simulink library "Pendel_Control"  (R2017b)
settings: Solver=VariableStepAuto  StartTime=0.0  StopTime=10.0  RelTol=1e-3
undefined symbols (not defined in the file): Angular2Linear, DiscIntNeverNeededParam, g, l, m, Ref_Bottom, Reset_Position_Bottom, SwitchAngle, U_Bottom
libraries: simulink x12, cstblocks x2
settings Model: Creator=BIROMED  LastModifiedBy=BIROMED

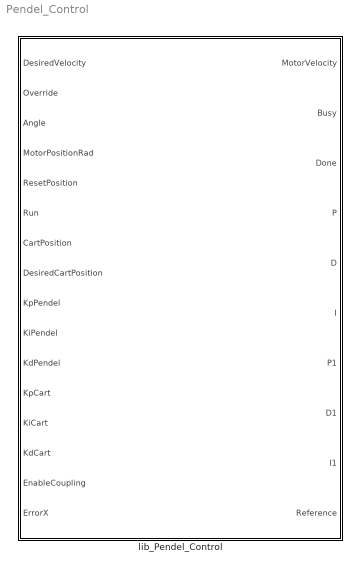
== system Pendel_Control ==
  lib_Pendel_Control : Subsystem

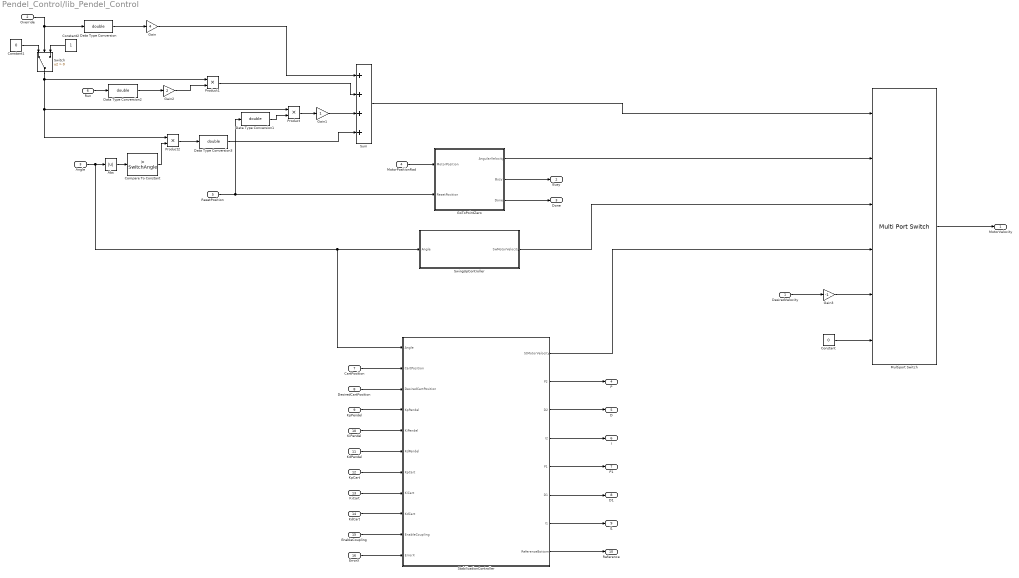
== system Pendel_Control/lib_Pendel_Control ==
  DesiredVelocity : Inport  OutDataTypeStr=double
  Override : Inport  Port=2  OutDataTypeStr=boolean
  Angle : Inport  Port=3
  MotorPositionRad : Inport  Port=4
  ResetPosition : Inport  Port=5  OutDataTypeStr=boolean
  Run : Inport  Port=6
  CartPosition : Inport  Port=7
  DesiredCartPosition : Inport  Port=8
  KpPendel : Inport  Port=9
  KiPendel : Inport  Port=10
  KdPendel : Inport  Port=11
  KpCart : Inport  Port=12  OutDataTypeStr=double
  KiCart : Inport  Port=13  OutDataTypeStr=double
  KdCart : Inport  Port=14  OutDataTypeStr=double
  EnableCoupling : Inport  Port=15  OutDataTypeStr=boolean
  ErrorX : Inport  Port=16  OutDataTypeStr=double
  Abs : Abs
  Compare To Constant : simulink/Logic and Bit Operations/Compare To Constant  relop=>  const=SwitchAngle  OutDataTypeStr=boolean
  Constant : Constant  Value=0
  Constant1 : Constant  Value=0
  Constant2 : Constant
  Data Type Conversion{,1..3} (4 alike) : DataTypeConversion  OutDataTypeStr=double
  Gain : Gain  Gain=4
  Gain1 : Gain
  Gain2 : Gain  Gain=2
  Gain3 : Gain  Gain=-1
  GoToPointZero : Subsystem
  Multiport Switch : MultiPortSwitch  Inputs=5
  Product : Product
  Product1 : Product
  Product2 : Product
  StabilizationController : Subsystem
  Sum : Sum  Inputs=++++
  SwingUpController : Subsystem
  Switch : Switch  Criteria=u2 > Threshold
  MotorVelocity : Outport
  Busy : Outport  Port=2  OutDataTypeStr=boolean
  Done : Outport  Port=3  OutDataTypeStr=boolean
  P : Outport  Port=4
  D : Outport  Port=5
  I : Outport  Port=6
  P1 : Outport  Port=7
  D1 : Outport  Port=8
  I1 : Outport  Port=9
  Reference : Outport  Port=10
  wires:
  KpCart/1 -> StabilizationController/7(KpCart)
  KpPendel/1 -> StabilizationController/4(KpPendel)
  EnableCoupling/1 -> StabilizationController/10(EnableCoupling)
  Data Type Conversion3/1 -> Sum/4
  KiPendel/1 -> StabilizationController/5(KiPendel)
  Data Type Conversion/1 -> Gain/1
  Gain3/1 -> Multiport Switch/5
  Product/1 -> Gain1/1
  StabilizationController/4(I2) -> I/1
  Gain2/1 -> Product1/2
  ResetPosition/1 -> GoToPointZero/2(ResetPosition), Data Type Conversion1/1
  Product1/1 -> Sum/2
  Override/1 -> Data Type Conversion/1, Switch/2
  GoToPointZero/2(Busy) -> Busy/1
  CartPosition/1 -> StabilizationController/2(CartPosition)
  StabilizationController/7(I1) -> I1/1
  Abs/1 -> Compare To Constant/1
  GoToPointZero/1(AngularVelocity) -> Multiport Switch/2
  DesiredCartPosition/1 -> StabilizationController/3(DesiredCartPosition)
  KiCart/1 -> StabilizationController/8(KiCart)
  Gain1/1 -> Sum/3
  Switch/1 -> Product1/1, Product2/1, Product/1
  StabilizationController/8(ReferenceBottom) -> Reference/1
  Product2/1 -> Data Type Conversion3/1
  Constant2/1 -> Switch/3
  Data Type Conversion2/1 -> Gain2/1
  Constant1/1 -> Switch/1
  Run/1 -> Data Type Conversion2/1
  Compare To Constant/1 -> Product2/2
  SwingUpController/1(SwMotorVelocity) -> Multiport Switch/3
  ErrorX/1 -> StabilizationController/11(ErrorX)
  Angle/1 -> StabilizationController/1(Angle), SwingUpController/1(Angle), Abs/1
  StabilizationController/6(D1) -> D1/1
  Sum/1 -> Multiport Switch/1
  StabilizationController/1(StMotorVelocity) -> Multiport Switch/4
  KdPendel/1 -> StabilizationController/6(KdPendel)
  Constant/1 -> Multiport Switch/6
  StabilizationController/3(D2) -> D/1
  StabilizationController/2(P2) -> P/1
  Gain/1 -> Sum/1
  DesiredVelocity/1 -> Gain3/1
  Multiport Switch/1 -> MotorVelocity/1
  KdCart/1 -> StabilizationController/9(KdCart)
  MotorPositionRad/1 -> GoToPointZero/1(MotorPosition)
  StabilizationController/5(P1) -> P1/1
  Data Type Conversion1/1 -> Product/2
  GoToPointZero/3(Done) -> Done/1

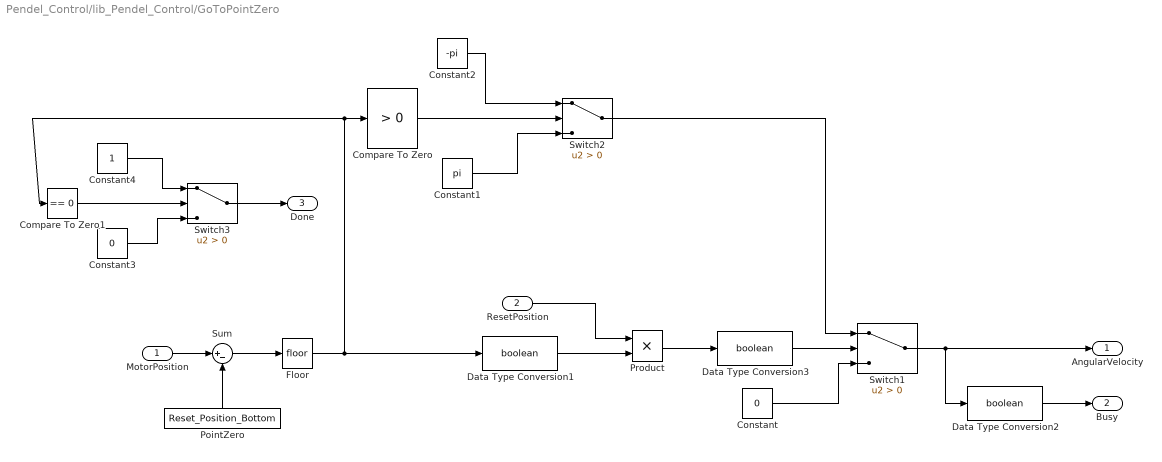
== system Pendel_Control/lib_Pendel_Control/GoToPointZero ==
  MotorPosition : Inport
  ResetPosition : Inport  Port=2
  Compare To Zero : simulink/Logic and Bit Operations/Compare To Zero  relop=>  OutDataTypeStr=boolean
  Compare To Zero1 : simulink/Logic and Bit Operations/Compare To Zero  relop===  OutDataTypeStr=boolean
  Constant : Constant  Value=0
  Constant1 : Constant  Value=pi
  Constant2 : Constant  Value=-pi
  Constant3 : Constant  Value=0
  Constant4 : Constant
  Data Type Conversion1 : DataTypeConversion  OutDataTypeStr=boolean
  Data Type Conversion2 : DataTypeConversion  OutDataTypeStr=boolean
  Data Type Conversion3 : DataTypeConversion  OutDataTypeStr=boolean
  Floor : Rounding
  PointZero : Constant  Value=Reset_Position_Bottom
  Product : Product
  Sum : Sum  Inputs=|+-
  Switch1 : Switch  Criteria=u2 > Threshold  OutDataTypeStr=double
  Switch2 : Switch  Criteria=u2 > Threshold
  Switch3 : Switch  Criteria=u2 > Threshold  OutDataTypeStr=boolean
  AngularVelocity : Outport
  Busy : Outport  Port=2
  Done : Outport  Port=3
  wires:
  Switch1/1 -> Data Type Conversion2/1, AngularVelocity/1
  PointZero/1 -> Sum/2
  Floor/1 -> Data Type Conversion1/1, Compare To Zero1/1, Compare To Zero/1
  MotorPosition/1 -> Sum/1
  Sum/1 -> Floor/1
  Constant/1 -> Switch1/3
  Compare To Zero/1 -> Switch2/2
  Constant1/1 -> Switch2/3
  Constant2/1 -> Switch2/1
  Switch2/1 -> Switch1/1
  Data Type Conversion2/1 -> Busy/1
  Data Type Conversion3/1 -> Switch1/2
  Constant3/1 -> Switch3/3
  Switch3/1 -> Done/1
  Constant4/1 -> Switch3/1
  Compare To Zero1/1 -> Switch3/2
  Product/1 -> Data Type Conversion3/1
  Data Type Conversion1/1 -> Product/2
  ResetPosition/1 -> Product/1

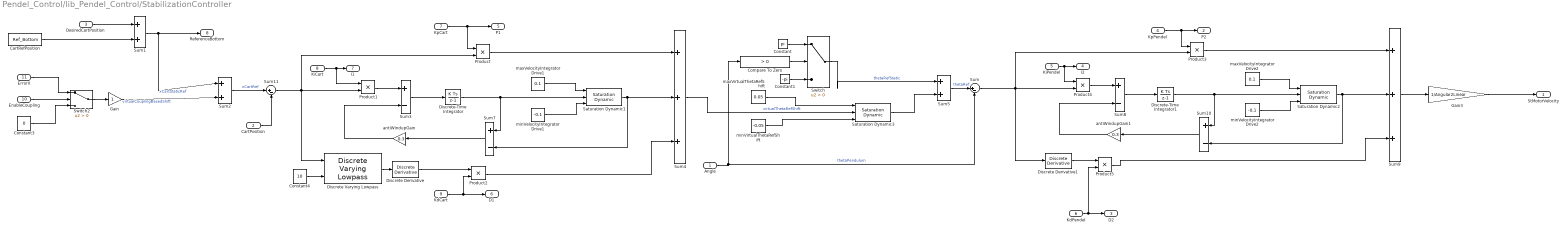
== system Pendel_Control/lib_Pendel_Control/StabilizationController ==
  Angle : Inport
  CartPosition : Inport  Port=2
  DesiredCartPosition : Inport  Port=3
  KpPendel : Inport  Port=4
  KiPendel : Inport  Port=5
  KdPendel : Inport  Port=6
  KpCart : Inport  Port=7
  KiCart : Inport  Port=8
  KdCart : Inport  Port=9
  EnableCoupling : Inport  Port=10
  ErrorX : Inport  Port=11
  CartRefPosition : Constant  Value=Ref_Bottom
  Compare To Zero : simulink/Logic and Bit Operations/Compare To Zero  relop=>  OutDataTypeStr=boolean
  Constant : Constant  Value=pi
  Constant1 : Constant  Value=-pi
  Constant3 : Constant  Value=0
  Constant4 : Constant  Value=10
  Discrete Derivative : simulink/Discrete/Discrete Derivative  gainval=1.0  ICPrevScaledInput=0.0  OutMin=[]  OutMax=[]  OutDataType=fixdt(1, 16)  OutScaling=2^-10  DoSatur=off
  Discrete Derivative1 : simulink/Discrete/Discrete Derivative  gainval=1.0  ICPrevScaledInput=0.0  OutMin=[]  OutMax=[]  OutDataType=fixdt(1, 16)  OutScaling=2^-10  DoSatur=off
  Discrete Varying Lowpass : cstblocks/Linear Parameter Varying/Discrete Varying Lowpass  N=1  w0=0  Ts=0.001
      settings: SourceProductName=Control System Toolbox  SourceProductBaseCode=CT
  Discrete-Time Integrator : DiscreteIntegrator  InitialConditionSetting=State (most efficient)  SampleTime=-1  ICPrevOutput=DiscIntNeverNeededParam  ICPrevScaledInput=DiscIntNeverNeededParam
  Discrete-Time Integrator1 : DiscreteIntegrator  InitialConditionSetting=State (most efficient)  SampleTime=-1  ICPrevOutput=DiscIntNeverNeededParam  ICPrevScaledInput=DiscIntNeverNeededParam
  Gain : Gain
  Gain3 : Gain  Gain=1/Angular2Linear
  Product{,1..5} (6 alike) : Product
  Saturation Dynamic1 : simulink/Discontinuities/Saturation Dynamic  OutMin=[]  OutMax=[]  OutDataTypeStr=Inherit: Same as second input  OutDataType=fixdt(1, 16)  OutScaling=2^-10  DoSatur=off
  Saturation Dynamic2 : simulink/Discontinuities/Saturation Dynamic  OutMin=[]  OutMax=[]  OutDataTypeStr=Inherit: Same as second input  OutDataType=fixdt(1, 16)  OutScaling=2^-10  DoSatur=off
  Saturation Dynamic3 : simulink/Discontinuities/Saturation Dynamic  OutMin=[]  OutMax=[]  OutDataTypeStr=Inherit: Same as second input  OutDataType=fixdt(1, 16)  OutScaling=2^-10  DoSatur=off
  Sum : Sum  Inputs=|+-
  Sum1 : Sum
  Sum{3,7..8,10} (4 alike) : Sum  Inputs=+-
  Sum11 : Sum  Inputs=|+-
  Sum2 : Sum  Inputs=|++
  Sum4 : Sum  Inputs=+++
  Sum5 : Sum  Inputs=|++
  Sum9 : Sum  Inputs=+++
  Switch : Switch  Criteria=u2 > Threshold
  Switch2 : Switch  Criteria=u2 > Threshold
  antiWindupGain : Gain  Gain=0.3
  antiWindupGain1 : Gain  Gain=0.3
  maxVelocityIntegratorDrive1 : Constant  Value=0.1
  maxVelocityIntegratorDrive2 : Constant  Value=0.1
  maxVirtualThetaRefShift : Constant  Value=0.05
  minVelocityIntegratorDrive1 : Constant  Value=-0.1
  minVelocityIntegratorDrive2 : Constant  Value=-0.1
  minVirtualThetaRefShift : Constant  Value=-0.05
  StMotorVelocity : Outport
  P2 : Outport  Port=2
  D2 : Outport  Port=3
  I2 : Outport  Port=4
  P1 : Outport  Port=5
  D1 : Outport  Port=6
  I1 : Outport  Port=7
  ReferenceBottom : Outport  Port=8
  wires:
  Sum5/1 -> Sum/1  "thetaRef"
  Compare To Zero/1 -> Switch/2
  CartPosition/1 -> Sum11/2
  KpPendel/1 -> Product3/1, P2/1
  KiPendel/1 -> Product4/1, I2/1
  KdPendel/1 -> Product5/2, D2/1
  KpCart/1 -> Product/1, P1/1
  KdCart/1 -> Product2/2, D1/1
  Gain3/1 -> StMotorVelocity/1
  Angle/1 -> Compare To Zero/1, Sum/2  "thetaPendulum"
  Constant/1 -> Switch/1
  Constant1/1 -> Switch/3
  KiCart/1 -> Product1/1, I1/1
  Sum9/1 -> Gain3/1
  Discrete-Time Integrator/1 -> Sum7/1, Saturation Dynamic1/2
  Sum11/1 -> Discrete Varying Lowpass/1, Product1/2, Product/2
  Sum3/1 -> Discrete-Time Integrator/1
  Sum7/1 -> antiWindupGain/1
  antiWindupGain/1 -> Sum3/2
  Saturation Dynamic1/1 -> Sum7/2, Sum4/2
  minVelocityIntegratorDrive1/1 -> Saturation Dynamic1/3
  Product1/1 -> Sum3/1
  maxVelocityIntegratorDrive1/1 -> Saturation Dynamic1/1
  Product/1 -> Sum4/1
  Product2/1 -> Sum4/3
  Sum4/1 -> Saturation Dynamic3/2  "virtualThetaRefShift"
  Product5/1 -> Sum9/3
  Product3/1 -> Sum9/1
  maxVelocityIntegratorDrive2/1 -> Saturation Dynamic2/1
  Product4/1 -> Sum8/1
  minVelocityIntegratorDrive2/1 -> Saturation Dynamic2/3
  Saturation Dynamic2/1 -> Sum10/2, Sum9/2
  antiWindupGain1/1 -> Sum8/2
  Sum10/1 -> antiWindupGain1/1
  Sum8/1 -> Discrete-Time Integrator1/1
  Sum/1 -> Product3/2, Discrete Derivative1/1, Product4/2
  Discrete-Time Integrator1/1 -> Saturation Dynamic2/2, Sum10/1
  Discrete Derivative/1 -> Product2/1
  Discrete Derivative1/1 -> Product5/1
  Discrete Varying Lowpass/1 -> Discrete Derivative/1
  Constant4/1 -> Discrete Varying Lowpass/2
  DesiredCartPosition/1 -> Sum1/1
  EnableCoupling/1 -> Switch2/2
  Sum1/1 -> Sum2/1, ReferenceBottom/1  "xCartStaticRef"
  CartRefPosition/1 -> Sum1/2
  ErrorX/1 -> Switch2/1
  Constant3/1 -> Switch2/3
  Switch2/1 -> Gain/1
  Gain/1 -> Sum2/2  "virtualCouplingBasedShift"
  Sum2/1 -> Sum11/1  "xCartRef"
  Switch/1 -> Sum5/1  "thetaRefStatic"
  maxVirtualThetaRefShift/1 -> Saturation Dynamic3/1
  minVirtualThetaRefShift/1 -> Saturation Dynamic3/3
  Saturation Dynamic3/1 -> Sum5/2

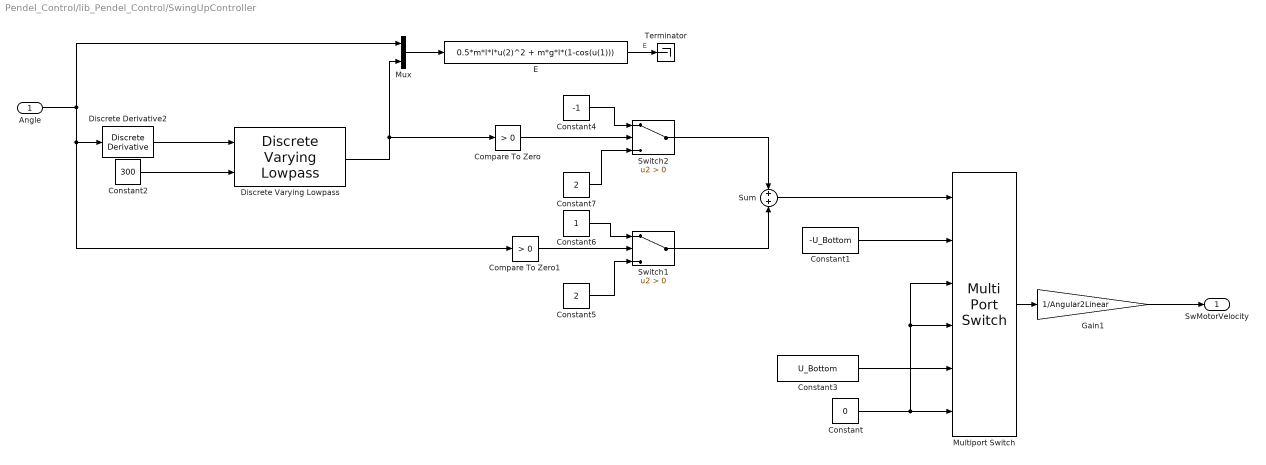
== system Pendel_Control/lib_Pendel_Control/SwingUpController ==
  Angle : Inport
  Compare To Zero : simulink/Logic and Bit Operations/Compare To Zero  relop=>  OutDataTypeStr=boolean
  Compare To Zero1 : simulink/Logic and Bit Operations/Compare To Zero  relop=>  OutDataTypeStr=boolean
  Constant : Constant  Value=0
  Constant1 : Constant  Value=-U_Bottom
  Constant2 : Constant  Value=300
  Constant3 : Constant  Value=U_Bottom
  Constant4 : Constant  Value=-1
  Constant5 : Constant  Value=2
  Constant6 : Constant
  Constant7 : Constant  Value=2
  Discrete Derivative2 : simulink/Discrete/Discrete Derivative  gainval=1.0  ICPrevScaledInput=0.0  OutMin=[]  OutMax=[]  OutDataType=fixdt(1, 16)  OutScaling=2^-10  DoSatur=off
  Discrete Varying Lowpass : cstblocks/Linear Parameter Varying/Discrete Varying Lowpass  N=1  w0=0  Ts=0.001
      settings: SourceProductName=Control System Toolbox  SourceProductBaseCode=CT
  E : Fcn  Expr=0.5*m*l*l*u(2)^2 + m*g*l*(1-cos(u(1)))
  Gain1 : Gain  Gain=1/Angular2Linear
  Multiport Switch : MultiPortSwitch  DataPortOrder=Specify indices  Inputs=5  DataPortIndices={0,1,3,4}  DataPortForDefault=Additional data port
  Mux : Mux  Inputs=2
  Sum : Sum
  Switch1 : Switch  Criteria=u2 > Threshold
  Switch2 : Switch  Criteria=u2 > Threshold
  Terminator : Terminator
  SwMotorVelocity : Outport
  wires:
  Mux/1 -> E/1
  Angle/1 -> Mux/1, Compare To Zero1/1, Discrete Derivative2/1
  Discrete Varying Lowpass/1 -> Compare To Zero/1, Mux/2
  Discrete Derivative2/1 -> Discrete Varying Lowpass/1
  Constant2/1 -> Discrete Varying Lowpass/2
  Gain1/1 -> SwMotorVelocity/1
  Compare To Zero/1 -> Switch2/2
  Constant4/1 -> Switch2/1
  Constant7/1 -> Switch2/3
  Constant1/1 -> Multiport Switch/2
  Constant3/1 -> Multiport Switch/5
  Multiport Switch/1 -> Gain1/1
  Sum/1 -> Multiport Switch/1
  Switch2/1 -> Sum/1
  Constant5/1 -> Switch1/3
  Constant6/1 -> Switch1/1
  Compare To Zero1/1 -> Switch1/2
  Switch1/1 -> Sum/2
  Constant/1 -> Multiport Switch/4, Multiport Switch/3, Multiport Switch/6
  E/1 -> Terminator/1  "E"
